simulink library "VsrLibEmissionsMeasUtils"  (R2019b)
settings: Solver=VariableStepAuto  StartTime=0.0  StopTime=10.0  RelTol=1e-3
settings Model: Creator=admin  LastModifiedBy=admin

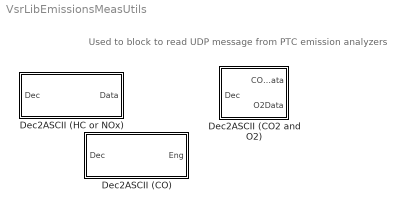
== system VsrLibEmissionsMeasUtils ==
  note: Used to block to read UDP message from PTC emission analyzers
  Dec2ASCII (CO) : Subsystem
  Dec2ASCII (CO2 and O2) : Subsystem
  Dec2ASCII (HC or NOx) : Subsystem

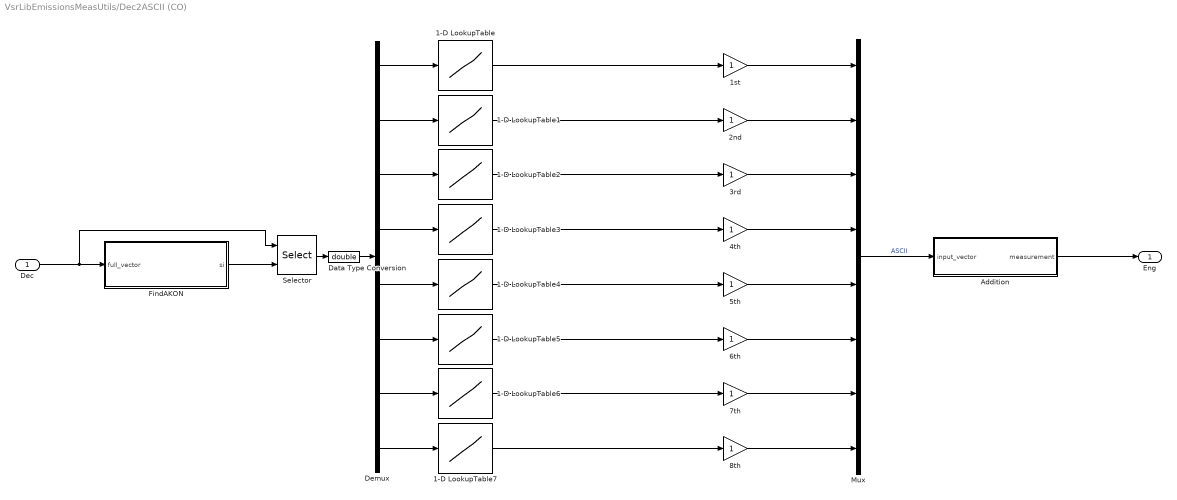
== system VsrLibEmissionsMeasUtils/Dec2ASCII (CO) ==
  Dec : Inport
  1-D LookupTable{,1..7} (8 alike) : Lookup_n-D  NumberOfTableDimensions=1  BreakpointsForDimension1=[48 49 50 51 52 53 54 55 56 57]  Table=[0 1 2 3 4 5 6 7 8 9]  InternalRulePriority=Speed  RndMeth=Simplest  InputSameDT=on
  1st : Gain
  2nd : Gain
  3rd : Gain
  4th : Gain
  5th : Gain
  6th : Gain
  7th : Gain
  8th : Gain
  Addition : MATLAB Function  TreatAsAtomicUnit=on
  Data Type Conversion : DataTypeConversion  OutDataTypeStr=double
  Demux : Demux  Outputs=8
  FindAKON : MATLAB Function  TreatAsAtomicUnit=on
  Mux : Mux  Inputs=8
  Selector : Selector  InputPortWidth=60  IndexOptions=Starting index (port)  Indices=[1 3]  OutputSizes=8
  Eng : Outport
  wires:
  Addition/1(measurement) -> Eng/1
  Dec/1 -> Selector/1, FindAKON/1(full_vector)
  FindAKON/1(si) -> Selector/2
  Demux/1 -> 1-D LookupTable/1
  Demux/7 -> 1-D LookupTable6/1
  Demux/3 -> 1-D LookupTable2/1
  Demux/5 -> 1-D LookupTable4/1
  Demux/4 -> 1-D LookupTable3/1
  Demux/2 -> 1-D LookupTable1/1
  Demux/6 -> 1-D LookupTable5/1
  1-D LookupTable5/1 -> 6th/1
  1-D LookupTable1/1 -> 2nd/1
  1-D LookupTable/1 -> 1st/1
  1-D LookupTable3/1 -> 4th/1
  1-D LookupTable6/1 -> 7th/1
  1-D LookupTable4/1 -> 5th/1
  1-D LookupTable2/1 -> 3rd/1
  1st/1 -> Mux/1
  2nd/1 -> Mux/2
  3rd/1 -> Mux/3
  4th/1 -> Mux/4
  5th/1 -> Mux/5
  6th/1 -> Mux/6
  7th/1 -> Mux/7
  Mux/1 -> Addition/1(input_vector)  "ASCII"
  Selector/1 -> Data Type Conversion/1
  Demux/8 -> 1-D LookupTable7/1
  1-D LookupTable7/1 -> 8th/1
  8th/1 -> Mux/8
  Data Type Conversion/1 -> Demux/1

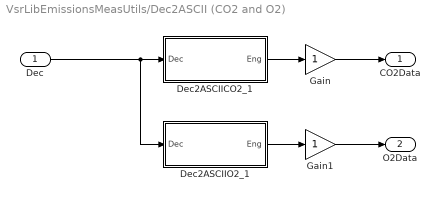
== system VsrLibEmissionsMeasUtils/Dec2ASCII (CO2 and O2) ==
  Dec : Inport
  Dec2ASCIICO2_1 : Subsystem
  Dec2ASCIIO2_1 : Subsystem
  Gain : Gain
  Gain1 : Gain
  CO2Data : Outport
  O2Data : Outport  Port=2
  wires:
  Dec2ASCIIO2_1/1(Eng) -> Gain1/1
  Dec/1 -> Dec2ASCIICO2_1/1(Dec), Dec2ASCIIO2_1/1(Dec)
  Dec2ASCIICO2_1/1(Eng) -> Gain/1
  Gain1/1 -> O2Data/1
  Gain/1 -> CO2Data/1

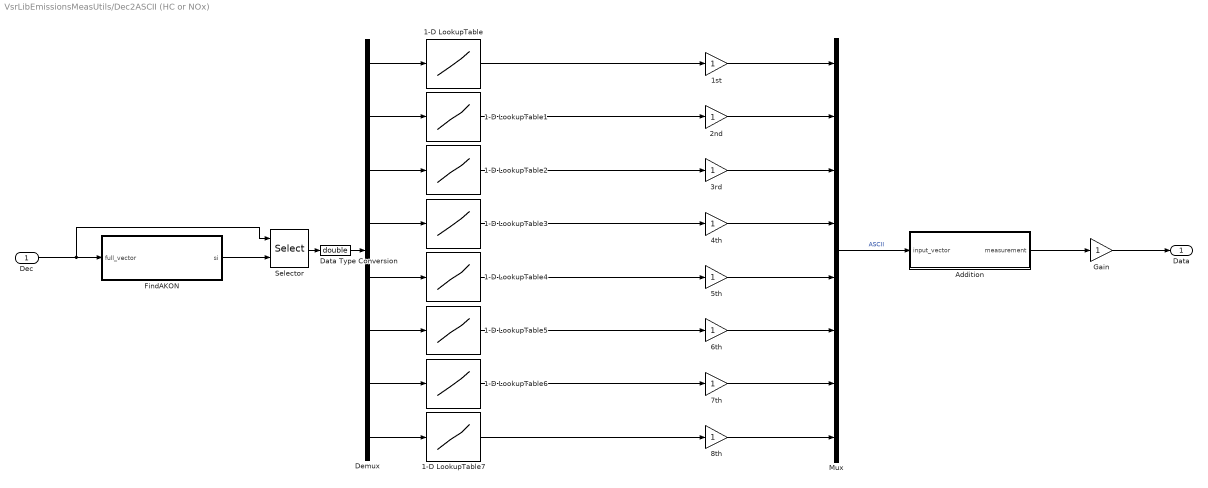
== system VsrLibEmissionsMeasUtils/Dec2ASCII (HC or NOx) ==
  Dec : Inport
  1-D LookupTable{,1..7} (8 alike) : Lookup_n-D  NumberOfTableDimensions=1  BreakpointsForDimension1=[48 49 50 51 52 53 54 55 56 57]  Table=[0 1 2 3 4 5 6 7 8 9]  InternalRulePriority=Speed  RndMeth=Simplest  InputSameDT=on
  1st : Gain
  2nd : Gain
  3rd : Gain
  4th : Gain
  5th : Gain
  6th : Gain
  7th : Gain
  8th : Gain
  Addition : MATLAB Function  TreatAsAtomicUnit=on
  Data Type Conversion : DataTypeConversion  OutDataTypeStr=double
  Demux : Demux  Outputs=8
  FindAKON : MATLAB Function  TreatAsAtomicUnit=on
  Gain : Gain
  Mux : Mux  Inputs=8
  Selector : Selector  InputPortWidth=80  IndexOptions=Starting index (port)  Indices=[1 3]  OutputSizes=8
  Data : Outport
  wires:
  Addition/1(measurement) -> Gain/1
  Dec/1 -> Selector/1, FindAKON/1(full_vector)
  FindAKON/1(si) -> Selector/2
  Demux/1 -> 1-D LookupTable/1
  Demux/7 -> 1-D LookupTable6/1
  Demux/3 -> 1-D LookupTable2/1
  Demux/5 -> 1-D LookupTable4/1
  Demux/4 -> 1-D LookupTable3/1
  Demux/2 -> 1-D LookupTable1/1
  Demux/6 -> 1-D LookupTable5/1
  1-D LookupTable5/1 -> 6th/1
  1-D LookupTable1/1 -> 2nd/1
  1-D LookupTable/1 -> 1st/1
  1-D LookupTable3/1 -> 4th/1
  1-D LookupTable6/1 -> 7th/1
  1-D LookupTable4/1 -> 5th/1
  1-D LookupTable2/1 -> 3rd/1
  1st/1 -> Mux/1
  2nd/1 -> Mux/2
  3rd/1 -> Mux/3
  4th/1 -> Mux/4
  5th/1 -> Mux/5
  6th/1 -> Mux/6
  7th/1 -> Mux/7
  Mux/1 -> Addition/1(input_vector)  "ASCII"
  Selector/1 -> Data Type Conversion/1
  Demux/8 -> 1-D LookupTable7/1
  1-D LookupTable7/1 -> 8th/1
  8th/1 -> Mux/8
  Data Type Conversion/1 -> Demux/1
  Gain/1 -> Data/1

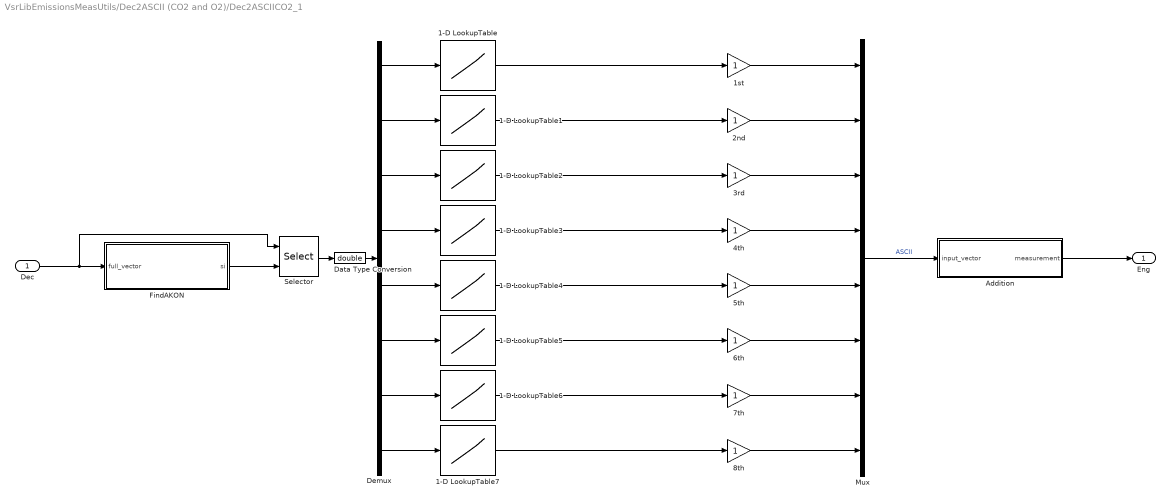
== system VsrLibEmissionsMeasUtils/Dec2ASCII (CO2 and O2)/Dec2ASCIICO2_1 ==
  Dec : Inport
  1-D LookupTable{,1..7} (8 alike) : Lookup_n-D  NumberOfTableDimensions=1  BreakpointsForDimension1=[48 49 50 51 52 53 54 55 56 57]  Table=[0 1 2 3 4 5 6 7 8 9]  InternalRulePriority=Speed  RndMeth=Simplest  InputSameDT=on
  1st : Gain
  2nd : Gain
  3rd : Gain
  4th : Gain
  5th : Gain
  6th : Gain
  7th : Gain
  8th : Gain
  Addition : MATLAB Function  TreatAsAtomicUnit=on
  Data Type Conversion : DataTypeConversion  OutDataTypeStr=double
  Demux : Demux  Outputs=8
  FindAKON : MATLAB Function  TreatAsAtomicUnit=on
  Mux : Mux  Inputs=8
  Selector : Selector  InputPortWidth=60  IndexOptions=Starting index (port)  Indices=[1 3]  OutputSizes=8
  Eng : Outport
  wires:
  Addition/1(measurement) -> Eng/1
  Dec/1 -> Selector/1, FindAKON/1(full_vector)
  FindAKON/1(si) -> Selector/2
  Demux/1 -> 1-D LookupTable/1
  Demux/7 -> 1-D LookupTable6/1
  Demux/3 -> 1-D LookupTable2/1
  Demux/5 -> 1-D LookupTable4/1
  Demux/4 -> 1-D LookupTable3/1
  Demux/2 -> 1-D LookupTable1/1
  Demux/6 -> 1-D LookupTable5/1
  1-D LookupTable5/1 -> 6th/1
  1-D LookupTable1/1 -> 2nd/1
  1-D LookupTable/1 -> 1st/1
  1-D LookupTable3/1 -> 4th/1
  1-D LookupTable6/1 -> 7th/1
  1-D LookupTable4/1 -> 5th/1
  1-D LookupTable2/1 -> 3rd/1
  1st/1 -> Mux/1
  2nd/1 -> Mux/2
  3rd/1 -> Mux/3
  4th/1 -> Mux/4
  5th/1 -> Mux/5
  6th/1 -> Mux/6
  7th/1 -> Mux/7
  Mux/1 -> Addition/1(input_vector)  "ASCII"
  Selector/1 -> Data Type Conversion/1
  Demux/8 -> 1-D LookupTable7/1
  1-D LookupTable7/1 -> 8th/1
  8th/1 -> Mux/8
  Data Type Conversion/1 -> Demux/1

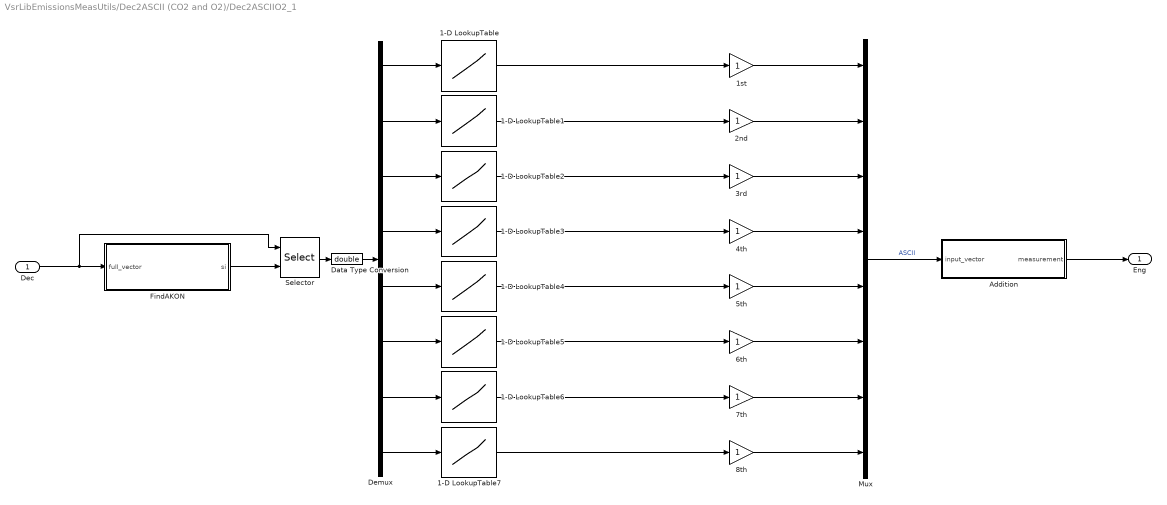
== system VsrLibEmissionsMeasUtils/Dec2ASCII (CO2 and O2)/Dec2ASCIIO2_1 ==
  Dec : Inport
  1-D LookupTable{,1..7} (8 alike) : Lookup_n-D  NumberOfTableDimensions=1  BreakpointsForDimension1=[48 49 50 51 52 53 54 55 56 57]  Table=[0 1 2 3 4 5 6 7 8 9]  InternalRulePriority=Speed  RndMeth=Simplest  InputSameDT=on
  1st : Gain
  2nd : Gain
  3rd : Gain
  4th : Gain
  5th : Gain
  6th : Gain
  7th : Gain
  8th : Gain
  Addition : MATLAB Function  TreatAsAtomicUnit=on
  Data Type Conversion : DataTypeConversion  OutDataTypeStr=double
  Demux : Demux  Outputs=8
  FindAKON : MATLAB Function  TreatAsAtomicUnit=on
  Mux : Mux  Inputs=8
  Selector : Selector  InputPortWidth=60  IndexOptions=Starting index (port)  Indices=[1 3]  OutputSizes=8
  Eng : Outport
  wires:
  Addition/1(measurement) -> Eng/1
  Dec/1 -> Selector/1, FindAKON/1(full_vector)
  FindAKON/1(si) -> Selector/2
  Demux/1 -> 1-D LookupTable/1
  Demux/7 -> 1-D LookupTable6/1
  Demux/3 -> 1-D LookupTable2/1
  Demux/5 -> 1-D LookupTable4/1
  Demux/4 -> 1-D LookupTable3/1
  Demux/2 -> 1-D LookupTable1/1
  Demux/6 -> 1-D LookupTable5/1
  1-D LookupTable5/1 -> 6th/1
  1-D LookupTable1/1 -> 2nd/1
  1-D LookupTable/1 -> 1st/1
  1-D LookupTable3/1 -> 4th/1
  1-D LookupTable6/1 -> 7th/1
  1-D LookupTable4/1 -> 5th/1
  1-D LookupTable2/1 -> 3rd/1
  1st/1 -> Mux/1
  2nd/1 -> Mux/2
  3rd/1 -> Mux/3
  4th/1 -> Mux/4
  5th/1 -> Mux/5
  6th/1 -> Mux/6
  7th/1 -> Mux/7
  Mux/1 -> Addition/1(input_vector)  "ASCII"
  Selector/1 -> Data Type Conversion/1
  Demux/8 -> 1-D LookupTable7/1
  1-D LookupTable7/1 -> 8th/1
  8th/1 -> Mux/8
  Data Type Conversion/1 -> Demux/1

== matlab function VsrLibEmissionsMeasUtils/Dec2ASCII (CO2 and O2)/Dec2ASCIICO2_1/Addition ==
  data: input_vector input; measurement output
function measurement = numassemble(input_vector)
if input_vector(1) == -3
    input_vector = input_vector(2:8);
    if input_vector(2) == -2
        if input_vector(1) == 0
            gains = [0;1.0E-01;1.0E-02;1.0E-03;1.0E-04;1.0E-05];
            inter = vertcat(input_vector(1),input_vector(3:7));
            measurement = sum(inter.*gains);
        else
            gains = [1;1.0E-01;1.0E-02;1.0E-03;1.0E-04;1.0E-05];
            inter = vertcat(input_vector(1),input_vector(3:7));
            measurement = sum(inter.*gains);
        end
    elseif input_vector(3) == -2
        gains = [1.0E+01;1;1.0E-01;1.0E-02;1.0E-03;1.0E-04];
        inter = vertcat(input_vector(1:2),input_vector(4:7));
        measurement = sum(inter.*gains);
    elseif input_vector(4) == -2
        gains = [1.0E+02;1.0E+01;1;1.0E-01;1.0E-02;1.0E-03];
        inter = vertcat(input_vector(1:3),input_vector(5:7));
        measurement = sum(inter.*gains);
    elseif input_vector(5) == -2
        gains = [1.0E+03;1.0E+02;1.0E+01;1;1.0E-01;1.0E-02];
        inter = vertcat(input_vector(1:4),input_vector(6:7));
        measurement = sum(inter.*gains);
    elseif input_vector(6) == -2
        gains = [1.0E+04;1.0E+03;1.0E+02;1.0E+01;1;1.0E-01];
        inter = vertcat(input_vector(1:5),input_vector(7));
        measurement = sum(inter.*gains);
    else
        gains = [1.0E+05;1.0E+04;1.0E+03;1.0E+02;1.0E+01;1;0];
        inter = vertcat(input_vector(1:7));
        measurement = sum(inter.*gains);
    end
    measurement = -1*measurement;
else
    if input_vector(2) == -2
        if input_vector(1) == 0
            gains = [0;1.0E-01;1.0E-02;1.0E-03;1.0E-04;1.0E-05;1.0E-06];
            inter = vertcat(input_vector(1),input_vector(3:8));
            measurement = sum(inter.*gains);
        else
            gains = [1;1.0E-01;1.0E-02;1.0E-03;1.0E-04;1.0E-05;1.0E-06];
            inter = vertcat(input_vector(1),input_vector(3:8));
            measurement = sum(inter.*gains);
        end
    elseif input_vector(3) == -2
        gains = [1.0E+01;1;1.0E-01;1.0E-02;1.0E-03;1.0E-04;1.0E-05];
        inter = vertcat(input_vector(1:2),input_vector(4:8));
        measurement = sum(inter.*gains);
    elseif input_vector(4) == -2
        gains = [1.0E+02;1.0E+01;1;1.0E-01;1.0E-02;1.0E-03;1.0E-04];
        inter = vertcat(input_vector(1:3),input_vector(5:8));
        measurement = sum(inter.*gains);
    elseif input_vector(5) == -2
        gains = [1.0E+03;1.0E+02;1.0E+01;1;1.0E-01;1.0E-02;1.0E-03];
        inter = vertcat(input_vector(1:4),input_vector(6:8));
        measurement = sum(inter.*gains);
    elseif input_vector(6) == -2
        gains = [1.0E+04;1.0E+03;1.0E+02;1.0E+01;1;1.0E-01;1.0E-02];
        inter = vertcat(input_vector(1:5),input_vector(7:8));
        measurement = sum(inter.*gains);
    elseif input_vector(7) == -2
        gains = [1.0E+05;1.0E+04;1.0E+03;1.0E+02;1.0E+01;1;1.0E-01];
        inter = vertcat(input_vector(1:6),input_vector(8));
        measurement = sum(inter.*gains);
    else
        gains = [1.0E+06;1.0E+05;1.0E+04;1.0E+03;1.0E+02;1.0E+01;1];
        measurement = sum(input_vector(1:7).*gains);
    end
end
    
return

== matlab function VsrLibEmissionsMeasUtils/Dec2ASCII (CO2 and O2)/Dec2ASCIIO2_1/Addition ==
  data: input_vector input; measurement output
function measurement = numassemble(input_vector)
if input_vector(1) == -3
    input_vector = input_vector(2:8);
    if input_vector(2) == -2
        if input_vector(1) == 0
            gains = [0;1.0E-01;1.0E-02;1.0E-03;1.0E-04;1.0E-05];
            inter = vertcat(input_vector(1),input_vector(3:7));
            measurement = sum(inter.*gains);
        else
            gains = [1;1.0E-01;1.0E-02;1.0E-03;1.0E-04;1.0E-05];
            inter = vertcat(input_vector(1),input_vector(3:7));
            measurement = sum(inter.*gains);
        end
    elseif input_vector(3) == -2
        gains = [1.0E+01;1;1.0E-01;1.0E-02;1.0E-03;1.0E-04];
        inter = vertcat(input_vector(1:2),input_vector(4:7));
        measurement = sum(inter.*gains);
    elseif input_vector(4) == -2
        gains = [1.0E+02;1.0E+01;1;1.0E-01;1.0E-02;1.0E-03];
        inter = vertcat(input_vector(1:3),input_vector(5:7));
        measurement = sum(inter.*gains);
    elseif input_vector(5) == -2
        gains = [1.0E+03;1.0E+02;1.0E+01;1;1.0E-01;1.0E-02];
        inter = vertcat(input_vector(1:4),input_vector(6:7));
        measurement = sum(inter.*gains);
    elseif input_vector(6) == -2
        gains = [1.0E+04;1.0E+03;1.0E+02;1.0E+01;1;1.0E-01];
        inter = vertcat(input_vector(1:5),input_vector(7));
        measurement = sum(inter.*gains);
    else
        gains = [1.0E+05;1.0E+04;1.0E+03;1.0E+02;1.0E+01;1;0];
        inter = vertcat(input_vector(1:7));
        measurement = sum(inter.*gains);
    end
    measurement = -1*measurement;
else
    if input_vector(2) == -2
        if input_vector(1) == 0
            gains = [0;1.0E-01;1.0E-02;1.0E-03;1.0E-04;1.0E-05;1.0E-06];
            inter = vertcat(input_vector(1),input_vector(3:8));
            measurement = sum(inter.*gains);
        else
            gains = [1;1.0E-01;1.0E-02;1.0E-03;1.0E-04;1.0E-05;1.0E-06];
            inter = vertcat(input_vector(1),input_vector(3:8));
            measurement = sum(inter.*gains);
        end
    elseif input_vector(3) == -2
        gains = [1.0E+01;1;1.0E-01;1.0E-02;1.0E-03;1.0E-04;1.0E-05];
        inter = vertcat(input_vector(1:2),input_vector(4:8));
        measurement = sum(inter.*gains);
    elseif input_vector(4) == -2
        gains = [1.0E+02;1.0E+01;1;1.0E-01;1.0E-02;1.0E-03;1.0E-04];
        inter = vertcat(input_vector(1:3),input_vector(5:8));
        measurement = sum(inter.*gains);
    elseif input_vector(5) == -2
        gains = [1.0E+03;1.0E+02;1.0E+01;1;1.0E-01;1.0E-02;1.0E-03];
        inter = vertcat(input_vector(1:4),input_vector(6:8));
        measurement = sum(inter.*gains);
    elseif input_vector(6) == -2
        gains = [1.0E+04;1.0E+03;1.0E+02;1.0E+01;1;1.0E-01;1.0E-02];
        inter = vertcat(input_vector(1:5),input_vector(7:8));
        measurement = sum(inter.*gains);
    elseif input_vector(7) == -2
        gains = [1.0E+05;1.0E+04;1.0E+03;1.0E+02;1.0E+01;1;1.0E-01];
        inter = vertcat(input_vector(1:6),input_vector(8));
        measurement = sum(inter.*gains);
    else
        gains = [1.0E+06;1.0E+05;1.0E+04;1.0E+03;1.0E+02;1.0E+01;1];
        measurement = sum(input_vector(1:7).*gains);
    end
end
    
return

== matlab function VsrLibEmissionsMeasUtils/Dec2ASCII (CO)/Addition ==
  data: input_vector input; measurement output
function measurement = numassemble(input_vector)
if input_vector(1) == -3
    input_vector = input_vector(2:8);
    if input_vector(2) == -2
        if input_vector(1) == 0
            gains = [0;1.0E-01;1.0E-02;1.0E-03;1.0E-04;1.0E-05];
            inter = vertcat(input_vector(1),input_vector(3:7));
            measurement = sum(inter.*gains);
        else
            gains = [1;1.0E-01;1.0E-02;1.0E-03;1.0E-04;1.0E-05];
            inter = vertcat(input_vector(1),input_vector(3:7));
            measurement = sum(inter.*gains);
        end
    elseif input_vector(3) == -2
        gains = [1.0E+01;1;1.0E-01;1.0E-02;1.0E-03;1.0E-04];
        inter = vertcat(input_vector(1:2),input_vector(4:7));
        measurement = sum(inter.*gains);
    elseif input_vector(4) == -2
        gains = [1.0E+02;1.0E+01;1;1.0E-01;1.0E-02;1.0E-03];
        inter = vertcat(input_vector(1:3),input_vector(5:7));
        measurement = sum(inter.*gains);
    elseif input_vector(5) == -2
        gains = [1.0E+03;1.0E+02;1.0E+01;1;1.0E-01;1.0E-02];
        inter = vertcat(input_vector(1:4),input_vector(6:7));
        measurement = sum(inter.*gains);
    elseif input_vector(6) == -2
        gains = [1.0E+04;1.0E+03;1.0E+02;1.0E+01;1;1.0E-01];
        inter = vertcat(input_vector(1:5),input_vector(7));
        measurement = sum(inter.*gains);
    else
        gains = [1.0E+05;1.0E+04;1.0E+03;1.0E+02;1.0E+01;1;0];
        inter = vertcat(input_vector(1:7));
        measurement = sum(inter.*gains);
    end
    measurement = -1*measurement;
else
    if input_vector(2) == -2
        if input_vector(1) == 0
            gains = [0;1.0E-01;1.0E-02;1.0E-03;1.0E-04;1.0E-05;1.0E-06];
            inter = vertcat(input_vector(1),input_vector(3:8));
            measurement = sum(inter.*gains);
        else
            gains = [1;1.0E-01;1.0E-02;1.0E-03;1.0E-04;1.0E-05;1.0E-06];
            inter = vertcat(input_vector(1),input_vector(3:8));
            measurement = sum(inter.*gains);
        end
    elseif input_vector(3) == -2
        gains = [1.0E+01;1;1.0E-01;1.0E-02;1.0E-03;1.0E-04;1.0E-05];
        inter = vertcat(input_vector(1:2),input_vector(4:8));
        measurement = sum(inter.*gains);
    elseif input_vector(4) == -2
        gains = [1.0E+02;1.0E+01;1;1.0E-01;1.0E-02;1.0E-03;1.0E-04];
        inter = vertcat(input_vector(1:3),input_vector(5:8));
        measurement = sum(inter.*gains);
    elseif input_vector(5) == -2
        gains = [1.0E+03;1.0E+02;1.0E+01;1;1.0E-01;1.0E-02;1.0E-03];
        inter = vertcat(input_vector(1:4),input_vector(6:8));
        measurement = sum(inter.*gains);
    elseif input_vector(6) == -2
        gains = [1.0E+04;1.0E+03;1.0E+02;1.0E+01;1;1.0E-01;1.0E-02];
        inter = vertcat(input_vector(1:5),input_vector(7:8));
        measurement = sum(inter.*gains);
    elseif input_vector(7) == -2
        gains = [1.0E+05;1.0E+04;1.0E+03;1.0E+02;1.0E+01;1;1.0E-01];
        inter = vertcat(input_vector(1:6),input_vector(8));
        measurement = sum(inter.*gains);
    else
        gains = [1.0E+06;1.0E+05;1.0E+04;1.0E+03;1.0E+02;1.0E+01;1];
        measurement = sum(input_vector(1:7).*gains);
    end
end
    
return

== matlab function VsrLibEmissionsMeasUtils/Dec2ASCII (CO)/FindAKON ==
  data: full_vector input; si output
function si = AKON(full_vector)
location = full_vector == 65;
[M,x] = max(location);
truncvec = full_vector(x:end);
newvec = truncvec == 32;
[M2,y] = max(newvec);
truncvec2 = truncvec(y+1:end);
newvec2 = truncvec2 == 32;
[M3,z] = max(newvec2);
si = (x+y+z);
return

== matlab function VsrLibEmissionsMeasUtils/Dec2ASCII (HC or NOx)/Addition ==
  data: input_vector input; measurement output
function measurement = numassemble(input_vector)
if input_vector(1) == -3
    input_vector = input_vector(2:8);
    if input_vector(2) == -2
        if input_vector(1) == 0
            gains = [0;1.0E-01;1.0E-02;1.0E-03;1.0E-04;1.0E-05];
            inter = vertcat(input_vector(1),input_vector(3:7));
            measurement = sum(inter.*gains);
        else
            gains = [1;1.0E-01;1.0E-02;1.0E-03;1.0E-04;1.0E-05];
            inter = vertcat(input_vector(1),input_vector(3:7));
            measurement = sum(inter.*gains);
        end
    elseif input_vector(3) == -2
        gains = [1.0E+01;1;1.0E-01;1.0E-02;1.0E-03;1.0E-04];
        inter = vertcat(input_vector(1:2),input_vector(4:7));
        measurement = sum(inter.*gains);
    elseif input_vector(4) == -2
        gains = [1.0E+02;1.0E+01;1;1.0E-01;1.0E-02;1.0E-03];
        inter = vertcat(input_vector(1:3),input_vector(5:7));
        measurement = sum(inter.*gains);
    elseif input_vector(5) == -2
        gains = [1.0E+03;1.0E+02;1.0E+01;1;1.0E-01;1.0E-02];
        inter = vertcat(input_vector(1:4),input_vector(6:7));
        measurement = sum(inter.*gains);
    elseif input_vector(6) == -2
        gains = [1.0E+04;1.0E+03;1.0E+02;1.0E+01;1;1.0E-01];
        inter = vertcat(input_vector(1:5),input_vector(7));
        measurement = sum(inter.*gains);
    else
        gains = [1.0E+05;1.0E+04;1.0E+03;1.0E+02;1.0E+01;1;0];
        inter = vertcat(input_vector(1:7));
        measurement = sum(inter.*gains);
    end
    measurement = -1*measurement;
else
    if input_vector(2) == -2
        if input_vector(1) == 0
            gains = [0;1.0E-01;1.0E-02;1.0E-03;1.0E-04;1.0E-05;1.0E-06];
            inter = vertcat(input_vector(1),input_vector(3:8));
            measurement = sum(inter.*gains);
        else
            gains = [1;1.0E-01;1.0E-02;1.0E-03;1.0E-04;1.0E-05;1.0E-06];
            inter = vertcat(input_vector(1),input_vector(3:8));
            measurement = sum(inter.*gains);
        end
    elseif input_vector(3) == -2
        gains = [1.0E+01;1;1.0E-01;1.0E-02;1.0E-03;1.0E-04;1.0E-05];
        inter = vertcat(input_vector(1:2),input_vector(4:8));
        measurement = sum(inter.*gains);
    elseif input_vector(4) == -2
        gains = [1.0E+02;1.0E+01;1;1.0E-01;1.0E-02;1.0E-03;1.0E-04];
        inter = vertcat(input_vector(1:3),input_vector(5:8));
        measurement = sum(inter.*gains);
    elseif input_vector(5) == -2
        gains = [1.0E+03;1.0E+02;1.0E+01;1;1.0E-01;1.0E-02;1.0E-03];
        inter = vertcat(input_vector(1:4),input_vector(6:8));
        measurement = sum(inter.*gains);
    elseif input_vector(6) == -2
        gains = [1.0E+04;1.0E+03;1.0E+02;1.0E+01;1;1.0E-01;1.0E-02];
        inter = vertcat(input_vector(1:5),input_vector(7:8));
        measurement = sum(inter.*gains);
    elseif input_vector(7) == -2
        gains = [1.0E+05;1.0E+04;1.0E+03;1.0E+02;1.0E+01;1;1.0E-01];
        inter = vertcat(input_vector(1:6),input_vector(8));
        measurement = sum(inter.*gains);
    else
        gains = [1.0E+06;1.0E+05;1.0E+04;1.0E+03;1.0E+02;1.0E+01;1];
        measurement = sum(input_vector(1:7).*gains);
    end
end
    
return

== matlab function VsrLibEmissionsMeasUtils/Dec2ASCII (CO2 and O2)/Dec2ASCIICO2_1/FindAKON ==
  data: full_vector input; si output
function si = AKON(full_vector)
location = full_vector == 65;
[M,x] = max(location);
truncvec = full_vector(x:end);
newvec = truncvec == 32;
[M2,y] = max(newvec);
si = (x+y);
return

== matlab function VsrLibEmissionsMeasUtils/Dec2ASCII (CO2 and O2)/Dec2ASCIIO2_1/FindAKON ==
  data: full_vector input; si output
function si = AKON(full_vector)
location = full_vector == 65;
[M,x] = max(location);
truncvec = full_vector(x:end);
newvec = truncvec == 32;
[M2,y] = max(newvec);
truncvec2 = truncvec(y+1:end);
newvec2 = truncvec2 == 32;
[M3,z] = max(newvec2);
truncvec3 = truncvec2(z+1:end);
newvec3 = truncvec3 == 32;
[M4,a] = max(newvec3);
si = (x+y+z+a);
return

== matlab function VsrLibEmissionsMeasUtils/Dec2ASCII (HC or NOx)/FindAKON ==
  data: full_vector input; si output
function si = AKON(full_vector)
location = full_vector == 65;
[M,x] = max(location);
truncvec = full_vector(x:end);
newvec = truncvec == 32;
[M2,y] = max(newvec);
si = (x+y);
return
